simulink model "V0"  (R2017b)
settings: Solver=FixedStepDiscrete  StartTime=0.0  StopTime=Ts_240p*20  RelTol=1e-3
InitFcn:
  | Ts = 1e-3;
  | Ts_240p = 402*324*Ts;
  | Ts_480p = 525*800*Ts;
undefined symbols (not defined in the file or in its folder): gray, Rec, SDTV
libraries: hdlsllib x8, visionhdlconversions x2, visionhdlio x2, visionconversions x1, visionanalysis x1, dspvision x1
settings Model: DataTypeOverride=Off  ModifiedByFormat=The MathWorks Inc.  NumberOfSteps=10  Creator=The MathWorks, Inc.  LastModifiedBy=The MathWorks Inc.
settings DataIOCC: LimitDataPoints=on  SaveFormat=Array  SaveOutput=off  SaveTime=off
settings OptimizationCC: BlockReduction=off  ConditionallyExecuteInputs=off  DefaultParameterBehavior=Inlined  LifeSpan=inf
settings DebuggingCC: AlgebraicLoopMsg=error  SolverPrmCheckMsg=warning  SingleTaskRateTransMsg=error  ParameterPrecisionLossMsg=none  AllowSymbolicDim=off  SFUnexpectedBacktrackingDiag=warning  SFNoUnconditionalDefaultTransitionDiag=warning  SFExecutionAtInitializationDiag=none  IntegerSaturationMsg=none
settings HardwareCC: ProdBitPerPointer=32  ProdBitPerSizeT=32  ProdBitPerPtrDiffT=32  ProdLargestAtomicFloat=None  ProdIntDivRoundTo=Undefined  ProdEndianess=Unspecified  ProdWordSize=32  ProdHWDeviceType=ASIC/FPGA->ASIC/FPGA  ProdEqTarget=off
settings ModelReferenceCC: PropagateSignalLabelsOutOfModel=off
settings CodeAppCC: StateflowObjectComments=on
settings GRTTargetCC: TargetLangStandard=C89/C90 (ANSI)  GeneratePreprocessorConditionals=Disable all
settings ConfigComp: CovMetricSettings=dw  CovHtmlReporting=on  CovSaveCumulativeToWorkspaceVar=on  CovSaveSingleToWorkspaceVar=on  CovShowResultsExplorer=off  CovExternalEMLEnable=off  CovSFcnEnable=off

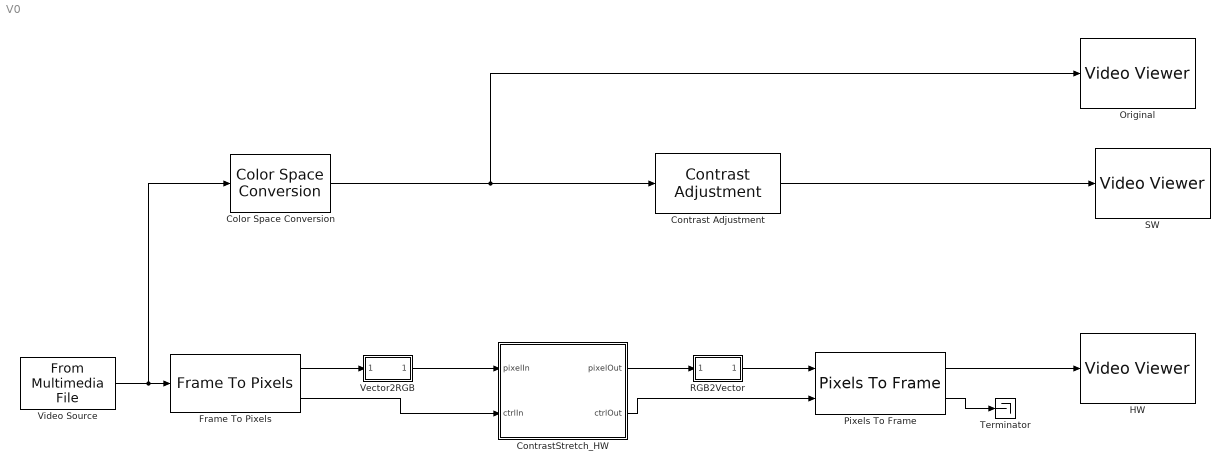
== system V0 ==
  Color Space Conversion : visionconversions/Color Space  Conversion  conversion=Obsolete  conversionActive=R'G'B' to intensity  wp_str=D65  rec=Rec. 601 (SDTV)  sys=1125/60/2:1  imagePorts=One multidimensional signal
      settings: SourceProductName=Computer Vision System Toolbox
  Contrast Adjustment : visionanalysis/Contrast Adjustment  methodInputRange=Range determined by saturating outlier pixels  rangeIn=[0 73]  fracSaturate=[0.5 0.5]  isBinNum=on  binNum=256  methodOutputRange=Full data type range  rangeOut=[0 255]  prod1Mode=Binary point scaling  prod1WordLength=32  prod1FracLength=16  prod2Mode=Binary point scaling  prod2WordLength=32  prod2FracLength=16  roundingMode=Floor  overflowMode=off
      settings: SourceProductName=Computer Vision System Toolbox  SourceProductBaseCode=VP
  ContrastStretch_HW : Subsystem  TreatAsAtomicUnit=on
  Frame To Pixels : visionhdlio/Frame To Pixels  NumComponents=3  VideoFormat=240p  ActivePixelsPerLine=32  ActiveVideoLines=18  TotalPixelsPerLine=42  TotalVideoLines=28  StartingActiveLine=6  FrontPorch=5  SampleTime=0
      settings: SourceProductName=Vision HDL Toolbox  SourceProductBaseCode=VT
  HW : VideoViewer  colormapValue=gray(256)  FigPos=[797.8 653.2 688 514.4]
  Original : VideoViewer  colormapValue=gray(256)  FigPos=[348.2 1220.4 688 509.6]
  Pixels To Frame : visionhdlio/Pixels To Frame  NumComponents=3  VideoFormat=240p  ActivePixelsPerLine=32  ActiveVideoLines=18  TotalPixelsPerLine=42  TotalVideoLines=28
      settings: SourceProductName=Vision HDL Toolbox  SourceProductBaseCode=VT
  RGB2Vector : Subsystem
  SW : VideoViewer  colormapValue=gray(256)  FigPos=[53.8 666 688 514.4]
  Terminator : Terminator
  Vector2RGB : Subsystem
  Video Source : dspvision/From Multimedia File  inputFilename=E:\RnD\Current_Projects\Musawwir\Frameworks\HW\Musawwir_HW_Zedboard\Custom_IP_Cores\Matlab\ContrastStretching\einstein_bright.jpg  loop=on  numPlays=inf  outputStreams=Video only  videoDataType=uint8  audioDataType=int16  inheritSampleTime=off  userDefinedSampleTime=Ts_240p  noAudioOutput=off  isIntensityVideo=off  fourcc=RGB  colorVideoFormat=One multidimensional signal  outputEOF=off  dataOrg=Column-major  audioFrameSize=1024  computeAudioFrameSize=off  outSamplingMode=Sample based
      settings: SourceProductBaseCode=VP
  wires:
  Pixels To Frame/2 -> Terminator/1
  Pixels To Frame/1 -> HW/1
  Vector2RGB/1(RGB) -> ContrastStretch_HW/1(pixelIn)
  ContrastStretch_HW/1(pixelOut) -> RGB2Vector/1(RGB)
  Video Source/1 -> Color Space Conversion/1, Frame To Pixels/1
  Frame To Pixels/2 -> ContrastStretch_HW/2(ctrlIn)
  Frame To Pixels/1 -> Vector2RGB/1(RGBVector)
  RGB2Vector/1(RGBVector) -> Pixels To Frame/1
  ContrastStretch_HW/2(ctrlOut) -> Pixels To Frame/2
  Contrast Adjustment/1 -> SW/1
  Color Space Conversion/1 -> Contrast Adjustment/1, Original/1

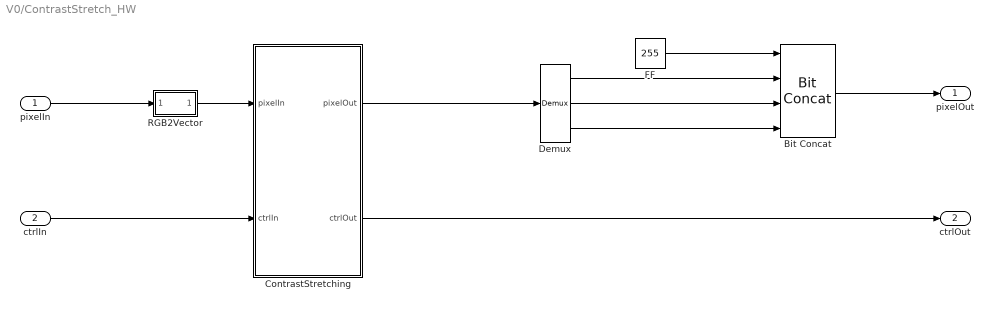
== system V0/ContrastStretch_HW ==
  pixelIn : Inport
  ctrlIn : Inport  Port=2
  Bit Concat : hdlsllib/Logic and Bit Operations/Bit Concat  numInputs=4
      settings: SourceProductName=HDL Coder  SourceProductBaseCode=HD
  ContrastStretching : Subsystem  TreatAsAtomicUnit=on
  Demux : Demux  Outputs=3
  FF : Constant  Value=255  OutDataTypeStr=uint8  SampleTime=Ts
  RGB2Vector : Subsystem
  pixelOut : Outport
  ctrlOut : Outport  Port=2
  wires:
  ctrlIn/1 -> ContrastStretching/2(ctrlIn)
  pixelIn/1 -> RGB2Vector/1(RGB)
  RGB2Vector/1(RGBVector) -> ContrastStretching/1(pixelIn)
  FF/1 -> Bit Concat/1
  Bit Concat/1 -> pixelOut/1
  Demux/3 -> Bit Concat/4
  Demux/2 -> Bit Concat/3
  Demux/1 -> Bit Concat/2
  ContrastStretching/2(ctrlOut) -> ctrlOut/1
  ContrastStretching/1(pixelOut) -> Demux/1

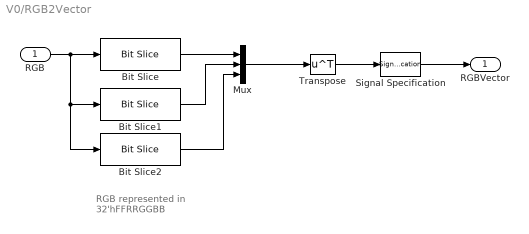
== system V0/RGB2Vector ==
  note: RGB represented in
      | 32'hFFRRGGBB
  RGB : Inport
  Bit Slice : hdlsllib/Logic and Bit Operations/Bit Slice  lidx=23  ridx=16
  Bit Slice1 : hdlsllib/Logic and Bit Operations/Bit Slice  lidx=15  ridx=8
  Bit Slice2 : hdlsllib/Logic and Bit Operations/Bit Slice  lidx=7  ridx=0
  Mux : Mux  Inputs=3
  Signal Specification : SignalSpecification
  Transpose : Math  Operator=transpose  SaturateOnIntegerOverflow=on
  RGBVector : Outport
  wires:
  Mux/1 -> Transpose/1
  Bit Slice/1 -> Mux/1
  Bit Slice2/1 -> Mux/3
  Bit Slice1/1 -> Mux/2
  RGB/1 -> Bit Slice2/1, Bit Slice1/1, Bit Slice/1
  Transpose/1 -> Signal Specification/1
  Signal Specification/1 -> RGBVector/1

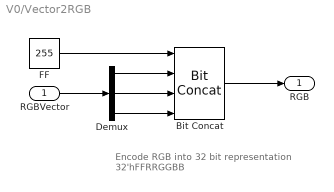
== system V0/Vector2RGB ==
  note: Encode RGB into 32 bit representation
      | 32'hFFRRGGBB
  RGBVector : Inport
  Bit Concat : hdlsllib/Logic and Bit Operations/Bit Concat  numInputs=4
      settings: SourceProductName=HDL Coder  SourceProductBaseCode=HD
  Demux : Demux  Outputs=3
  FF : Constant  Value=255  OutDataTypeStr=uint8  SampleTime=Ts
  RGB : Outport
  wires:
  Bit Concat/1 -> RGB/1
  RGBVector/1 -> Demux/1
  FF/1 -> Bit Concat/1
  Demux/1 -> Bit Concat/2
  Demux/2 -> Bit Concat/3
  Demux/3 -> Bit Concat/4

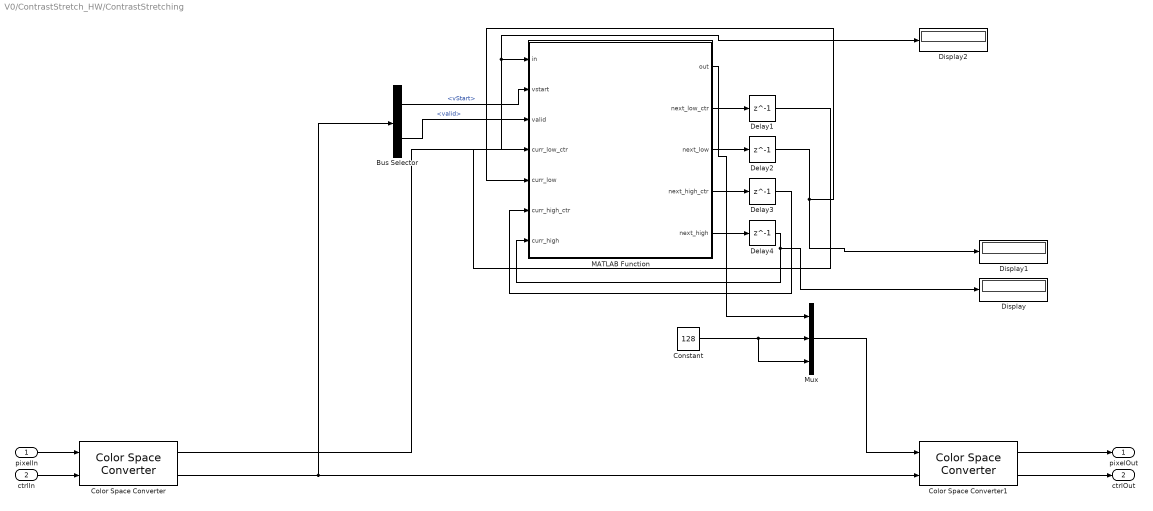
== system V0/ContrastStretch_HW/ContrastStretching ==
  pixelIn : Inport
  ctrlIn : Inport  Port=2
  Bus Selector : BusSelector  OutputSignals=vStart,valid
  Color Space Converter : visionhdlconversions/Color Space Converter  Conversion=RGB to intensity  ConversionStandard=Rec. 601 (SDTV)  ScanningStandard=1250/50/2:1  SimulateUsing=Code generation
      settings: SourceProductName=Vision HDL Toolbox  SourceProductBaseCode=VT
  Color Space Converter1 : visionhdlconversions/Color Space Converter  Conversion=YCbCr to RGB  ConversionStandard=Rec. 601 (SDTV)  ScanningStandard=1250/50/2:1  SimulateUsing=Code generation
      settings: SourceProductName=Vision HDL Toolbox  SourceProductBaseCode=VT
  Constant : Constant  Value=128  OutDataTypeStr=uint8
  Delay1 : Delay  DelayLength=1  InitialCondition=0
  Delay2 : Delay  DelayLength=1  InitialCondition=10
  Delay3 : Delay  DelayLength=1  InitialCondition=0
  Delay4 : Delay  DelayLength=1  InitialCondition=255
  Display : Display
  Display1 : Display
  Display2 : Display
  MATLAB Function : MATLAB Function  TreatAsAtomicUnit=on
  Mux : Mux  Inputs=3
  pixelOut : Outport
  ctrlOut : Outport  Port=2
  wires:
  pixelIn/1 -> Color Space Converter/1
  ctrlIn/1 -> Color Space Converter/2
  Color Space Converter1/1 -> pixelOut/1
  Color Space Converter1/2 -> ctrlOut/1
  Color Space Converter/1 -> Display2/1, MATLAB Function/1(in)
  Color Space Converter/2 -> Bus Selector/1, Color Space Converter1/2
  Mux/1 -> Color Space Converter1/1
  MATLAB Function/2(next_low_ctr) -> Delay1/1
  Delay1/1 -> MATLAB Function/4(curr_low_ctr)
  MATLAB Function/3(next_low) -> Delay2/1
  Delay2/1 -> Display1/1, MATLAB Function/5(curr_low)
  Bus Selector/1 -> MATLAB Function/2(vstart)  "<vStart>"
  Bus Selector/2 -> MATLAB Function/3(valid)  "<valid>"
  MATLAB Function/1(out) -> Mux/1
  Constant/1 -> Mux/3, Mux/2
  MATLAB Function/4(next_high_ctr) -> Delay3/1
  MATLAB Function/5(next_high) -> Delay4/1
  Delay4/1 -> Display/1, MATLAB Function/7(curr_high)
  Delay3/1 -> MATLAB Function/6(curr_high_ctr)

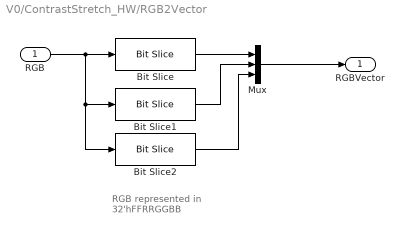
== system V0/ContrastStretch_HW/RGB2Vector ==
  note: RGB represented in
      | 32'hFFRRGGBB
  RGB : Inport
  Bit Slice : hdlsllib/Logic and Bit Operations/Bit Slice  lidx=23  ridx=16
  Bit Slice1 : hdlsllib/Logic and Bit Operations/Bit Slice  lidx=15  ridx=8
  Bit Slice2 : hdlsllib/Logic and Bit Operations/Bit Slice  lidx=7  ridx=0
  Mux : Mux  Inputs=3
  RGBVector : Outport
  wires:
  Bit Slice/1 -> Mux/1
  Bit Slice2/1 -> Mux/3
  Bit Slice1/1 -> Mux/2
  RGB/1 -> Bit Slice2/1, Bit Slice1/1, Bit Slice/1
  Mux/1 -> RGBVector/1

== matlab function V0/ContrastStretch_HW/ContrastStretching/MATLAB Function ==
  data: in input; vstart input; valid input; out output uint8 size=[1,1]; curr_low_ctr input single; next_low_ctr output single; curr_low input single; next_low output single; curr_high_ctr input single; curr_high input single; next_high_ctr output single; next_high output single
function [out, next_low_ctr, next_low, next_high_ctr, next_high] = lower_limt(in, vstart, valid, curr_low_ctr, curr_low, curr_high_ctr, curr_high)
% next_low = single(0);

prob_limit = 0.5*(320*240)/100;
step = 10;

if(vstart==1)
    next_low_ctr = single(0);
else
    if((in<curr_low)&(valid==1))
        next_low_ctr = curr_low_ctr + 1;
    else
        next_low_ctr = curr_low_ctr;
    end
end

if(vstart==1)
    if(curr_low_ctr<=prob_limit)%150*curr_low)
        next_low = curr_low + step;
    else
%         if(curr_low>0)
            next_low = curr_low - step;
%         else
%             next_low = curr_low;
%         end
    end
else
    next_low = curr_low;
end

if(vstart==1)
    next_high_ctr = single(0);
else
    if((in>curr_high)&(valid==1))
        next_high_ctr = curr_high_ctr + 1;
    else
        next_high_ctr = curr_high_ctr;
    end
end

if(vstart==1)
    if(curr_high_ctr<=prob_limit)%150*(255-curr_high))
        next_high = curr_high - step;
    else
%         if(curr_low>0)
            next_high = curr_high + step;
%         else
%             next_low = curr_low;
%         end
    end
else
    next_high = curr_high;
end


% if(in<curr_high)
%     next_high = curr_high - (0.0001220703125);
% else
%     next_high = curr_high + (0.0001220703125);
% end

low = curr_low;
high = curr_high;%255;
in_ = single(in);
out_ = (in_-low)*255/(high-low);
out = uint8(out_);
